simulink model "longmen2"  (R2023b)
settings: Solver=VariableStepAuto  StartTime=0.0  StopTime=10.0  RelTol=1e-3
settings Model: Creator=asus  LastModifiedBy=asus

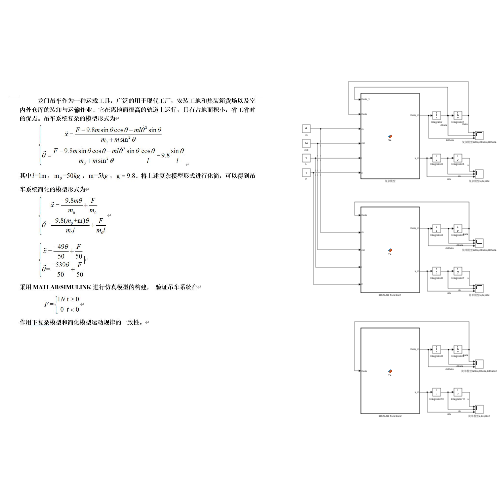
[thumbnail: Simulink's stored preview of the top-level diagram]
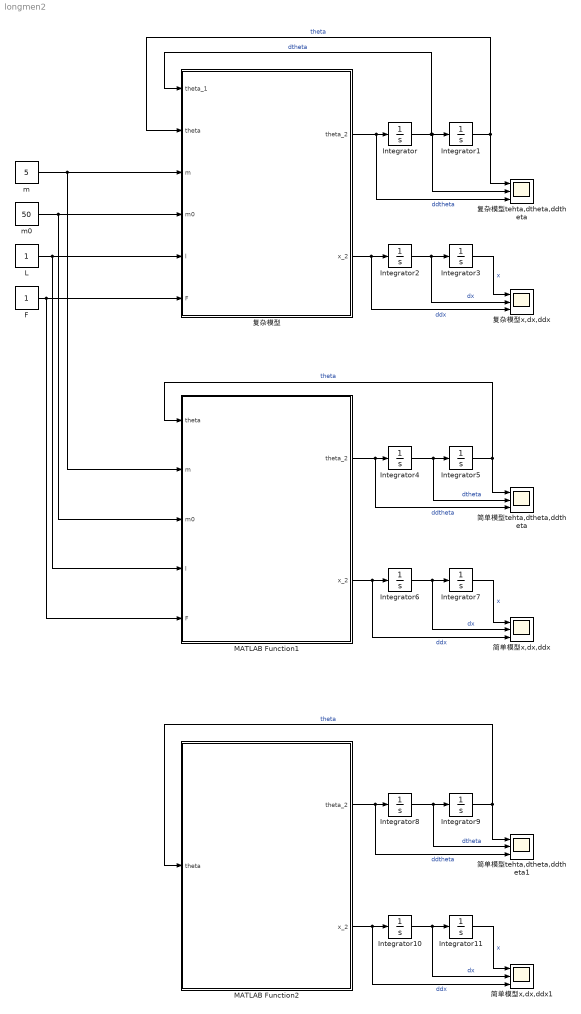
== system longmen2 ==
  F : Constant
  Integrator{,1..11} (12 alike) : Integrator
  L : Constant
  MATLAB Function1 : MATLAB Function  TreatAsAtomicUnit=on
  MATLAB Function2 : MATLAB Function  TreatAsAtomicUnit=on
  m : Constant  Value=5
  m0 : Constant  Value=50
  复杂模型 : MATLAB Function  TreatAsAtomicUnit=on
  复杂模型tehta,dtheta,ddtheta : Scope  NumInputPorts=3
  复杂模型x,dx,ddx : Scope  NumInputPorts=3
  简单模型tehta,dtheta,ddtheta : Scope  NumInputPorts=3
  简单模型tehta,dtheta,ddtheta1 : Scope  NumInputPorts=3
  简单模型x,dx,ddx : Scope  NumInputPorts=3
  简单模型x,dx,ddx1 : Scope  NumInputPorts=3
  wires:
  m/1 -> MATLAB Function1/2(m), 复杂模型/3(m)
  m0/1 -> MATLAB Function1/3(m0), 复杂模型/4(m0)
  F/1 -> MATLAB Function1/5(F), 复杂模型/6(F)
  L/1 -> MATLAB Function1/4(l), 复杂模型/5(l)
  复杂模型/1(theta_2) -> 复杂模型tehta,dtheta,ddtheta/3, Integrator/1  "ddtheta"
  Integrator/1 -> 复杂模型/1(theta_1), 复杂模型tehta,dtheta,ddtheta/2, Integrator1/1  "dtheta"
  Integrator1/1 -> 复杂模型tehta,dtheta,ddtheta/1, 复杂模型/2(theta)  "theta"
  复杂模型/2(x_2) -> 复杂模型x,dx,ddx/3, Integrator2/1  "ddx"
  Integrator2/1 -> 复杂模型x,dx,ddx/2, Integrator3/1  "dx"
  MATLAB Function1/1(theta_2) -> 简单模型tehta,dtheta,ddtheta/3, Integrator4/1  "ddtheta"
  Integrator4/1 -> 简单模型tehta,dtheta,ddtheta/2, Integrator5/1  "dtheta"
  Integrator5/1 -> 简单模型tehta,dtheta,ddtheta/1, MATLAB Function1/1(theta)  "theta"
  Integrator6/1 -> 简单模型x,dx,ddx/2, Integrator7/1  "dx"
  MATLAB Function1/2(x_2) -> 简单模型x,dx,ddx/3, Integrator6/1  "ddx"
  Integrator3/1 -> 复杂模型x,dx,ddx/1  "x"
  Integrator7/1 -> 简单模型x,dx,ddx/1  "x"
  Integrator11/1 -> 简单模型x,dx,ddx1/1  "x"
  MATLAB Function2/2(x_2) -> Integrator10/1, 简单模型x,dx,ddx1/3  "ddx"
  Integrator10/1 -> Integrator11/1, 简单模型x,dx,ddx1/2  "dx"
  Integrator9/1 -> MATLAB Function2/1(theta), 简单模型tehta,dtheta,ddtheta1/1  "theta"
  Integrator8/1 -> Integrator9/1, 简单模型tehta,dtheta,ddtheta1/2  "dtheta"
  MATLAB Function2/1(theta_2) -> Integrator8/1, 简单模型tehta,dtheta,ddtheta1/3  "ddtheta"

== matlab function longmen2/MATLAB Function1 ==
  data: theta_2 output; x_2 output; theta input; m input; m0 input; l input; F input
function [theta_2,x_2] = fcn(theta,m,m0,l,F)

% x_2m = m0 + m*(sin(theta))^2;
% x_2z = F - 9.8*m*sin(theta)*cos(theta) - m*l*(theta_1^2)*sin(theta);
% x_2=x_2z / x_2m;
% 
% theta_2 = x_2*cos(theta)/l - 9.8*sin(theta)/l;

x_2 = -9.8*m*theta/m0 + F/m0;
theta_2 = -9.8*(m+m0)*theta/(m0*l) + F/(m0*l);

== matlab function longmen2/复杂模型 ==
  data: theta_1 input; theta_2 output; x_2 output; theta input; m input; m0 input; l input; F input
function [theta_2,x_2] = fcn(theta_1,theta,m,m0,l,F)

x_2m = m0 + m*(sin(theta))^2;
x_2z = F - 9.8*m*sin(theta)*cos(theta) - m*l*(theta_1^2)*sin(theta);
x_2=x_2z / x_2m;

theta_2 = x_2*cos(theta)/l - 9.8*sin(theta)/l;

== matlab function longmen2/MATLAB Function2 ==
  data: theta_2 output; x_2 output; theta input
function [theta_2,x_2] = fcn(theta)

x_2 = -49*theta/50 + 1/50;
theta_2 = -539*theta/50 + 1/50;
